simulink model "igbt_power_inverter_det"  (R2014a)
settings: Solver=ode23tb  StartTime=0.0  StopTime=1  RelTol=1e-4
PreLoadFcn:
  | Ts = 1e-6;
  | Tc = 1e-4;
StartFcn:
  | tic;
StopFcn:
  | toc;
undefined symbols (not defined in the file or in its folder): D1, Delta, DiscIntNeverNeededParam
libraries: powerlib x10, powerlib_meascontrol x4, simulink x2
settings Model: Creator=cosorio  LastModifiedBy=cosorio
settings DataIOCC: SaveOutput=off  DSMLogging=off  SaveTime=off
settings DebuggingCC: SolverPrmCheckMsg=none

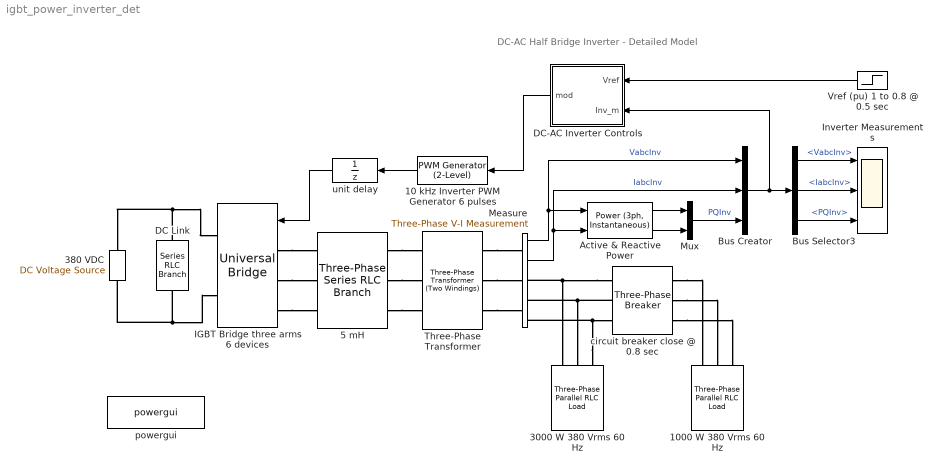
== system igbt_power_inverter_det ==
  note: DC-AC Half Bridge Inverter - Detailed Model
  10 kHz Inverter PWM Generator 6 pulses : powerlib_meascontrol/Pulse & Signal Generators/PWM Generator (2-Level)  ModulatorType=Three-phase bridge (6 pulses)  ModulatorMode=Unsynchronized  nF=27  Fc=1e04  ModulatingSignals=off  m=0.8  Freq=60  Phase=0  Ts=Ts
  1000 W 380 Vrms 60 Hz : powerlib/Elements/Three-Phase Parallel RLC Load  LConnTagsString=A|B|C  Configuration=Y (grounded)  NominalVoltage=380  NominalFrequency=60  ActivePower=1000  InductivePower=0  CapacitivePower=0  Measurements=None  LoadType=constant Z
  3000 W 380 Vrms 60 Hz : powerlib/Elements/Three-Phase Parallel RLC Load  LConnTagsString=A|B|C  Configuration=Y (grounded)  NominalVoltage=380  NominalFrequency=60  ActivePower=3000  InductivePower=0  CapacitivePower=0  Measurements=None  LoadType=constant Z
  380 VDC : powerlib/Electrical Sources/DC Voltage Source  Amplitude=380  Measurements=None
  "5 mH " : powerlib/Elements/Three-Phase Series RLC Branch  LConnTagsString=A|B|C  RConnTagsString=A|B|C  BranchType=RL  Resistance=0.25  Inductance=5e-3  Capacitance=1.0  Measurements=None
  Active & Reactive Power : powerlib_meascontrol/Measurements/Power (3ph, Instantaneous)
  Bus Creator : BusCreator  Inputs=3
  Bus Selector3 : BusSelector  OutputSignals=VabcInv,IabcInv,PQInv
  DC Link : powerlib/Elements/Series RLC Branch  LConnTagsString=__new0  RConnTagsString=__new0  BranchType=RC  Resistance=0.25  Inductance=30e-6  SetiL0=off  InitialCurrent=0  Capacitance=1200e-6  Setx0=on  InitialVoltage=380  Measurements=None
  DC-AC Inverter Controls : Subsystem  TreatAsAtomicUnit=on  SystemSampleTime=Tc
  IGBT Bridge three arms 6 devices : powerlib/Power Electronics/Universal Bridge  Arms=3  SnubberResistance=1e5  SnubberCapacitance=inf  Device=IGBT / Diodes  Ron=1e-4  Lon=0  ForwardVoltages="[  0  0  ]"  ForwardVoltage=0  GTOparameters=[ 10e-6 , 20e-6 ]  IGBTparameters=[ 1e-6 , 2e-6 ]  Measurements=None  Measurements_2=None  converterType=Rectifier
  Inverter Measurements : Scope  NumInputPorts=3
      settings: YMin=-400~-10~-1000  YMax=400~10~4000  SaveName=InverterData
  Measure : powerlib/Measurements/Three-Phase V-I Measurement  VoltageMeasurement=phase-to-ground  SetLabelV=off  LabelV=V1  Vpu=off  VpuLL=off  CurrentMeasurement=yes  SetLabelI=off  LabelI=I1  Ipu=off  Pbase=3000*sqrt(3)  Vbase=380  OutputType=Magnitude  PhasorSimulation=off  PSBequivalent=0
  Mux : Mux  Inputs=2
  Three-Phase Transformer : powerlib/Elements/Three-Phase Transformer (Two Windings)  Winding1Connection=Delta (D1)  UNITS=pu  NominalPower=[3000 , 60 ]  Winding1=[110 , 0.002 , 0.08 ]  Winding2Connection=Yg  Winding2=[380 , 0.002 , 0.08 ]  SetSaturation=off  Rm=500  Lm=500  Saturation=[ 0,0 ; 0.0024,1.2 ; 1.0,1.52 ]  Hysteresis=off  DataFile='hysteresis'  SetInitialFlux=off  InitialFluxes=[ 0.8 , -0.8 , 0.7 ]  Measurements=None  MoreParameters=off  BreakLoop=off  DataType=off  TransfoNumber=1
  Vref (pu) 1 to 0.8 @ 0.5 sec : Step  Time=0.5  Before=1  After=0.8  SampleTime=1e-4
  circuit breaker close @ 0.8 sec : powerlib/Elements/Three-Phase Breaker  InitialState=open  SwitchA=on  SwitchB=on  SwitchC=on  SwitchTimes=[0.8]  External=off  BreakerResistance=0.001  SnubberResistance=1e6  SnubberCapacitance=inf  Measurements=None
  powergui : powerlib/powergui  Priority=1  SimulationMode=Continuous  SolverType=Tustin  SampleTime=Ts  frequency=60  SPID=off  DisableSnubberDevices=off  DisableRonSwitches=off  DisableVfSwitches=off  SwTol=0  Interpol=off  DisplayEquations=off  Ts=0  methode=off  frequencyindice=0  Pbase=100e6  ErrMax=1e-4  Iterations=50  UnitsV=kV  UnitsW=MW  FunctionMessages=off  echomessages=off  HookPort=off  EnableUseOfTLC=off  x0status=blocks  RestoreLinks=warning  ResistiveCurrentMeasurement=off  Frange=[0:2:500]  Ylog=off  Xlog=on  ShowGrid=off  save=off  variable=ZData  structure=InverterData  ZoomFFT=off  StartTime=0.1  cycles=4  DisplayStyle=1  fundamental=60  FreqAxis=on  MaxFrequency=24000  frequencyindicesteady=1  RmsSteady=1  display=off
  unit delay : UnitDelay  SampleTime=Ts
  wires:
  Vref (pu) 1 to 0.8 @ 0.5 sec/1 -> DC-AC Inverter Controls/1(Vref)
  Bus Selector3/1 -> Inverter Measurements/1  "<VabcInv>"
  Bus Selector3/2 -> Inverter Measurements/2  "<IabcInv>"
  Bus Selector3/3 -> Inverter Measurements/3  "<PQInv>"
  10 kHz Inverter PWM Generator 6 pulses/1 -> unit delay/1
  DC-AC Inverter Controls/1(mod) -> 10 kHz Inverter PWM Generator 6 pulses/1
  Measure/1 -> Active & Reactive Power/1, Bus Creator/1  "VabcInv"
  Measure/2 -> Active & Reactive Power/2, Bus Creator/2  "IabcInv"
  unit delay/1 -> IGBT Bridge three arms 6 devices/1
  Mux/1 -> Bus Creator/3  "PQInv"
  Active & Reactive Power/1 -> Mux/1
  Active & Reactive Power/2 -> Mux/2
  Bus Creator/1 -> DC-AC Inverter Controls/2(Inv_m), Bus Selector3/1
  connections:
  circuit breaker close @ 0.8 sec/RConn1 -- 1000 W 380 Vrms 60 Hz/LConn1
  circuit breaker close @ 0.8 sec/RConn2 -- 1000 W 380 Vrms 60 Hz/LConn2
  circuit breaker close @ 0.8 sec/RConn3 -- 1000 W 380 Vrms 60 Hz/LConn3
  DC Link/LConn1 -- IGBT Bridge three arms 6 devices/RConn1 -- 380 VDC/RConn1
  IGBT Bridge three arms 6 devices/RConn2 -- DC Link/RConn1 -- 380 VDC/LConn1
  IGBT Bridge three arms 6 devices/LConn1 -- "5 mH "/LConn1
  IGBT Bridge three arms 6 devices/LConn2 -- "5 mH "/LConn2
  IGBT Bridge three arms 6 devices/LConn3 -- "5 mH "/LConn3
  circuit breaker close @ 0.8 sec/LConn1 -- 3000 W 380 Vrms 60 Hz/LConn1 -- Measure/RConn1
  circuit breaker close @ 0.8 sec/LConn2 -- 3000 W 380 Vrms 60 Hz/LConn2 -- Measure/RConn2
  3000 W 380 Vrms 60 Hz/LConn3 -- circuit breaker close @ 0.8 sec/LConn3 -- Measure/RConn3
  "5 mH "/RConn1 -- Three-Phase Transformer/LConn1
  "5 mH "/RConn2 -- Three-Phase Transformer/LConn2
  "5 mH "/RConn3 -- Three-Phase Transformer/LConn3
  Three-Phase Transformer/RConn3 -- Measure/LConn3
  Three-Phase Transformer/RConn2 -- Measure/LConn2
  Three-Phase Transformer/RConn1 -- Measure/LConn1

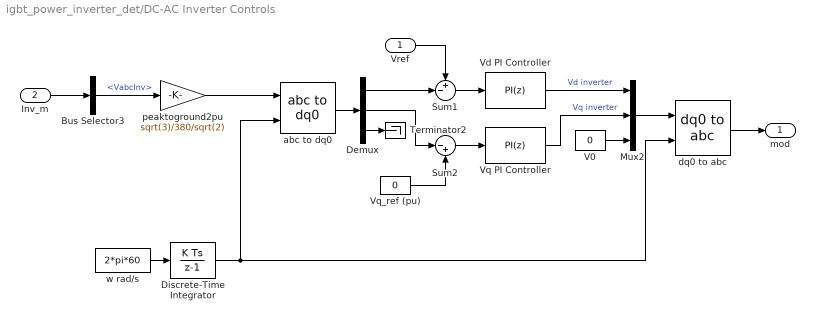
== system igbt_power_inverter_det/DC-AC Inverter Controls ==
  Vref : Inport  SampleTime=Tc
  Inv_m : Inport  Port=2  SampleTime=Tc
  Bus Selector3 : BusSelector  OutputSignals=VabcInv
  Demux : Demux  Outputs=3
  Discrete-Time Integrator : DiscreteIntegrator  SampleTime=Tc  ICPrevOutput=DiscIntNeverNeededParam  ICPrevScaledInput=DiscIntNeverNeededParam
  Mux2 : Mux  Inputs=3
  Sum1 : Sum  Inputs=+-|  SaturateOnIntegerOverflow=on  InputSameDT=on  OutDataTypeStr=Inherit: Same as first input
  Sum2 : Sum  Inputs=|-+  SaturateOnIntegerOverflow=on  InputSameDT=on  OutDataTypeStr=Inherit: Same as first input
  Terminator2 : Terminator
  V0 : Constant  Value=0
  Vd PI Controller : simulink/Continuous/PID Controller  Controller=PI  TimeDomain=Discrete-time  SampleTime=Tc  IntegratorMethod=Forward Euler  FilterMethod=Forward Euler  Form=Parallel  P=0.1  I=100  D=0  N=100  InitialConditionSource=internal  InitialConditionForIntegrator=0  InitialConditionForFilter=0  ExternalReset=none  LimitOutput=on  UpperSaturationLimit=1  LowerSaturationLimit=0  LinearizeAsGain=on  AntiWindupMode=clamping  Kb=1  TrackingMode=off  Kt=1  PParamMin=[]  PParamMax=[]  IParamMin=[]  IParamMax=[]  DParamMin=[]  DParamMax=[]  NParamMin=[]  NParamMax=[]  KbParamMin=[]  KbParamMax=[]  KtParamMin=[]  KtParamMax=[]  POutMin=[]  POutMax=[]  IOutMin=[]  IOutMax=[]  DOutMin=[]  DOutMax=[]  NOutMin=[]  NOutMax=[]  KbOutMin=[]  KbOutMax=[]  KtOutMin=[]  KtOutMax=[]  IntegratorOutMin=[]  IntegratorOutMax=[]  FilterOutMin=[]  FilterOutMax=[]  SumOutMin=[]  SumOutMax=[]  SumI1OutMin=[]  SumI1OutMax=[]  SumI2OutMin=[]  SumI2OutMax=[]  SumI3OutMin=[]  SumI3OutMax=[]  SumDOutMin=[]  SumDOutMax=[]  SaturationOutMin=[]  SaturationOutMax=[]  IntegratorContinuousStateAttributes=''  IntegratorStateMustResolveToSignalObject=off  IntegratorRTWStateStorageClass=Auto  FilterContinuousStateAttributes=''  FilterStateMustResolveToSignalObject=off  FilterRTWStateStorageClass=Auto
  Vq PI Controller : simulink/Continuous/PID Controller  Controller=PI  TimeDomain=Discrete-time  SampleTime=Tc  IntegratorMethod=Forward Euler  FilterMethod=Forward Euler  Form=Parallel  P=0.1  I=100  D=0  N=100  InitialConditionSource=internal  InitialConditionForIntegrator=0  InitialConditionForFilter=0  ExternalReset=none  LimitOutput=on  UpperSaturationLimit=1  LowerSaturationLimit=-1  LinearizeAsGain=on  AntiWindupMode=clamping  Kb=1  TrackingMode=off  Kt=1  PParamMin=[]  PParamMax=[]  IParamMin=[]  IParamMax=[]  DParamMin=[]  DParamMax=[]  NParamMin=[]  NParamMax=[]  KbParamMin=[]  KbParamMax=[]  KtParamMin=[]  KtParamMax=[]  POutMin=[]  POutMax=[]  IOutMin=[]  IOutMax=[]  DOutMin=[]  DOutMax=[]  NOutMin=[]  NOutMax=[]  KbOutMin=[]  KbOutMax=[]  KtOutMin=[]  KtOutMax=[]  IntegratorOutMin=[]  IntegratorOutMax=[]  FilterOutMin=[]  FilterOutMax=[]  SumOutMin=[]  SumOutMax=[]  SumI1OutMin=[]  SumI1OutMax=[]  SumI2OutMin=[]  SumI2OutMax=[]  SumI3OutMin=[]  SumI3OutMax=[]  SumDOutMin=[]  SumDOutMax=[]  SaturationOutMin=[]  SaturationOutMax=[]  IntegratorContinuousStateAttributes=''  IntegratorStateMustResolveToSignalObject=off  IntegratorRTWStateStorageClass=Auto  FilterContinuousStateAttributes=''  FilterStateMustResolveToSignalObject=off  FilterRTWStateStorageClass=Auto
  Vq_ref (pu) : Constant  Value=0
  abc to dq0 : powerlib_meascontrol/Transformations/abc to dq0  Alignment=90 degrees behind phase A axis
  dq0 to abc : powerlib_meascontrol/Transformations/dq0 to abc  Alignment=90 degrees behind phase A axis
  peaktoground2pu : Gain  Gain=sqrt(3)/380/sqrt(2)
  w rad/s : Constant  Value=2*pi*60
  mod : Outport
  wires:
  Bus Selector3/1 -> peaktoground2pu/1  "<VabcInv>"
  Inv_m/1 -> Bus Selector3/1
  dq0 to abc/1 -> mod/1
  Demux/3 -> Terminator2/1
  Vref/1 -> Sum1/1
  Demux/1 -> Sum1/2
  V0/1 -> Mux2/3
  Vq PI Controller/1 -> Mux2/2  "Vq inverter"
  Demux/2 -> Sum2/1
  Vq_ref (pu)/1 -> Sum2/2
  Sum2/1 -> Vq PI Controller/1
  abc to dq0/1 -> Demux/1
  peaktoground2pu/1 -> abc to dq0/1
  Sum1/1 -> Vd PI Controller/1
  Mux2/1 -> dq0 to abc/1
  Discrete-Time Integrator/1 -> dq0 to abc/2, abc to dq0/2
  Vd PI Controller/1 -> Mux2/1  "Vd inverter"
  w rad/s/1 -> Discrete-Time Integrator/1
